simulink model "PubIfDecisionTOS_MDL"  (R2020b)
settings: configuration reference "DspaceConfig" (kept outside this file)
PostLoadFcn:
  | if any(exist('dsrtsu_mdlpostloadfcn', 'file') ~= 0), dsrtsu_mdlpostloadfcn('Execute', bdroot); end
InitFcn:
  | , if any(exist('dsmpb_private', 'file') ~= 0), dsmpb_private('dsmpb_mdlclblib', 'Init', bdroot); end,
undefined symbols (not defined in the file or in its folder): C_TOS_ACCEgoRAxletoFbumplength_m, C_TOS_ACCTargetFront_Flag, C_TOS_AEBJAPedObjDxThre_Val, C_TOS_AEBJAPedObjDyThre_Val, C_TOS_AEBJATargetSize_Val, C_TOS_AEBJAVehObjDxThre_Val, C_TOS_AEBJAVehObjDyThre_Val, C_TOS_AEBJuncPedTargetSize_Val, C_TOS_AEBLatObjDxThre_Val, C_TOS_AEBLatPedDyThre_Val, C_TOS_AEBLatTargetSize_Val, C_TOS_AEBLongTargetInEgoFront_Flag, C_TOS_axAbsGround_Parameter, C_TOS_CameraConfirmedFlag, C_TOS_CNsubjWidth, C_TOS_CurrentLaneCoreMinWidth_Val, C_TOS_CutInProb_Val_Zero, C_TOS_CutOutProb_Val_Zero, C_TOS_D2R_Val, C_TOS_DefaultValueObjectToCenterLine_dy, C_TOS_EgoCarWidth_Val, C_TOS_EgoDxRefPoint_m, C_TOS_EgoRAxletoFbumplength_m, C_TOS_HalfWidthVehicle_Con, C_TOS_HWA_CurrentLaneFlag, C_TOS_HWA_LeftLaneFlag, C_TOS_HWA_MovingDir_Vaild, C_TOS_HWA_MovState_Vaild, C_TOS_HWA_RightLaneFlag, C_TOS_LaneLineCourseErrorFront, C_TOS_LaneLineCourseErrorRear, C_TOS_MotorbikeDefaultWidth_m, C_TOS_NumberOfEffectiveTargets, C_TOS_Obj_Age_Val, C_TOS_Objdx_Constraint_Val, C_TOS_ObjectDefaultWidth_m, C_TOS_ObjInCurrentLane_Val, C_TOS_ObjInCurrentLaneValid, C_TOS_ObjInLeftLaneValid, C_TOS_ObjInRightLaneValid, C_TOS_ObjNotInCurrentLane_Val, C_TOS_ObjNotREElementType, C_TOS_ObjPredictDis_dy_ConstantVal_Zeros, C_TOS_ObjToCenterLine_ConstantVal_Zeros, C_TOS_OFMObjIDInvilad_Val, C_TOS_PIL_LatDisCons_Val_zero, C_TOS_PIL_ObjectCutInFlag_b, C_TOS_PIL_ObjectCutOutFlag_b, C_TOS_PIL_ObjLaneProb_al_Val, C_TOS_PP_ObjFusType_FC_Confirm_b, C_TOS_PP_ObjFusType_FC_FR_Confirm_b, C_TOS_PP_ObjFusType_FR_Confirm_b, C_TOS_RE_80BoolDefault_Val, C_TOS_RE_80Single181Default_Val, C_TOS_RE_80Single255Default_Val, C_TOS_RE_80Uint8Default_Val, C_TOS_RE_D2R, C_TOS_RE_D_180_Val, C_TOS_RE_InvalidObjectID_Val, C_TOS_RE_InvalidTargetChainDir_Val ... (+142)
libraries: simulink x1650, TOS_LIB x361, canfdmsglib x14
(part 46 of 69)

== system PubIfDecisionTOS_MDL/TOS_20201112/TOS_2012080320/TOS/AEB/TOS_AEBJunct1105/AEBJunc_Object_Condition/AEBJA_TargetCondition/TOS_AEBJunc_TargetsCondition/AEBJunc_VehTargetCondition/AEBJunc_VehTargetObjectTypeFlag ==
  ObjectType : Inport
  AEBJunc_VehTarget_ID_K1 : Inport  Port=2
  ObjectID : Inport  Port=3
  AEBJunc_VehTargetObjectTypeAborDly : Subsystem
  Compare To Constant3 : simulink/Logic and Bit Operations/Compare To Constant  relop===  const=OFM_OBJ_TYPE_E.CAR  OutDataTypeStr=boolean
      settings: AttributesFormatString=%<const>
  Compare To Constant4 : simulink/Logic and Bit Operations/Compare To Constant  relop===  const=OFM_OBJ_TYPE_E.TRUCK  OutDataTypeStr=boolean
      settings: AttributesFormatString=%<const>
  Data Type Conversion : DataTypeConversion  OutDataTypeStr=Enum: OFM_OBJ_TYPE_E
  Logical Operator3 : Logic  Operator=OR  AllPortsSameDT=off  OutDataTypeStr=boolean
  AEBJunc_VehTargetObjectTypeFlag : Outport
  wires:
  Logical Operator3/1 -> AEBJunc_VehTargetObjectTypeAborDly/3(TOS_AEBJunc_VehObjectType)
  ObjectType/1 -> Data Type Conversion/1
  Data Type Conversion/1 -> Compare To Constant3/1, Compare To Constant4/1
  Compare To Constant3/1 -> Logical Operator3/1
  Compare To Constant4/1 -> Logical Operator3/2
  AEBJunc_VehTarget_ID_K1/1 -> AEBJunc_VehTargetObjectTypeAborDly/1(AEBJunc_VehTarget_ID_K1)
  ObjectID/1 -> AEBJunc_VehTargetObjectTypeAborDly/2(ObjectID)
  AEBJunc_VehTargetObjectTypeAborDly/1(TOS_AEBJunc_VehObjectTypeFilt) -> AEBJunc_VehTargetObjectTypeFlag/1

== system PubIfDecisionTOS_MDL/TOS_20201112/TOS_2012080320/TOS/AEB/TOS_AEBJunct1105/AEBJunc_Object_Condition/AEBJA_TargetCondition/TOS_AEBJunc_TargetsCondition/AEBJunc_VehTargetCondition/Subsystem ==
  Object_MovingState : Inport
  Compare To Constant1 : simulink/Logic and Bit Operations/Compare To Constant  relop===  const=OFM_OBJ_MOVINGSTATE_E.MOVING  OutDataTypeStr=boolean
      settings: AttributesFormatString=%<const> = 2
  Compare To Constant2 : simulink/Logic and Bit Operations/Compare To Constant  relop===  const=OFM_OBJ_MOVINGSTATE_E.MOVING_SLOWLY  OutDataTypeStr=boolean
      settings: AttributesFormatString=%<const> = 5
  Data Type Conversion : DataTypeConversion  OutDataTypeStr=Enum: OFM_OBJ_MOVINGSTATE_E
  Logical Operator1 : Logic  Operator=OR  AllPortsSameDT=off  OutDataTypeStr=boolean
  TOS_AEBJuncVehTargetMovStateFlg : Outport
  wires:
  Compare To Constant1/1 -> Logical Operator1/1
  Logical Operator1/1 -> TOS_AEBJuncVehTargetMovStateFlg/1
  Compare To Constant2/1 -> Logical Operator1/2
  Object_MovingState/1 -> Data Type Conversion/1
  Data Type Conversion/1 -> Compare To Constant2/1, Compare To Constant1/1

== system PubIfDecisionTOS_MDL/TOS_20201112/TOS_2012080320/TOS/AEB/TOS_AEBJunct1105/AEBJunc_Object_Condition/AEBJA_TargetCondition/TOS_AEBJunc_TargetsCondition/AEBJunc_VehTargetCondition/TOS_AEBJunc_VehTargetMoveDir ==
  Object_Dx : Inport
  PP_ObjMovingDirSignalProcessing : Inport  Port=2
  Object_HeadingAngle : Inport  Port=3
  Object_VX : Inport  Port=4
  Object_VY : Inport  Port=5
  VIE_EgoVelocity : Inport  Port=6
  axvRefMs2 : Inport  Port=7
  Abs{,1..3} (4 alike) : Abs
  Add{,2..4} (4 alike) : Sum
  Add1 : Sum  Inputs=+-
  Compare To Constant : simulink/Logic and Bit Operations/Compare To Constant  relop=<  const=P_TOS_OncomingTarget_VxabsOffset_val  OutDataTypeStr=boolean
      settings: AttributesFormatString=%<const> = -0.7m/s
  Compare To Constant1 : simulink/Logic and Bit Operations/Compare To Constant  relop=>  const=P_TOS_CrossingTargetVyvThre_val  OutDataTypeStr=boolean
      settings: AttributesFormatString=%<const>
  Compare To Constant16 : simulink/Logic and Bit Operations/Compare To Constant  relop=>  const=P_TOS_ObjLatCroYawAngMaxThre_Val  OutDataTypeStr=boolean
      settings: AttributesFormatString=P_TOS_ObjLatCroYawAngMaxThre_Val = 135
  Compare To Constant2 : simulink/Logic and Bit Operations/Compare To Constant  relop===  const=ObjectMovingOrientation_E.OnComingDir  OutDataTypeStr=boolean
      settings: AttributesFormatString=%<const>
  Compare To Constant3 : simulink/Logic and Bit Operations/Compare To Constant  relop=>  const=P_TOS_ObjOncomingYawAngMaxThre_Val  OutDataTypeStr=boolean
      settings: AttributesFormatString=P_TOS_ObjOncomingYawAngMaxThre_Val = 180
  Compare To Constant4 : simulink/Logic and Bit Operations/Compare To Constant  relop=<  const=0  OutDataTypeStr=boolean
  Constant : Constant  Value=C_TOS_StepTime_Val
  Constant1 : Constant  Value=C_TOS_StepTime_Val
  Constant2 : Constant  Value=P_TOS_OncomingVehDxChangeOffset_Val
  Data Type Conversion2 : DataTypeConversion  OutDataTypeStr=Enum: ObjectMovingOrientation_E
  Gain : Gain  Gain=1/2
  Gain1 : Gain  Gain=1/2
  Logical Operator : Logic  Operator=OR  Inputs=4  AllPortsSameDT=off  OutDataTypeStr=boolean
  Logical Operator{1..3,10} (4 alike) : Logic  AllPortsSameDT=off  OutDataTypeStr=boolean
  Math Function : Math  Operator=square  SaturateOnIntegerOverflow=on
  Product : Product
  Product1 : Product
  Relational Operator : RelationalOperator  Operator=>  OutDataTypeStr=boolean  RndMeth=Simplest
  Unit Delay{,1..3} (4 alike) : UnitDelay  InitialCondition=255  SampleTime=-1  HasFrameUpgradeWarning=on
  TOS_AEBJuncVehTargetMovDirFlg : Outport
  wires:
  Logical Operator/1 -> TOS_AEBJuncVehTargetMovDirFlg/1
  VIE_EgoVelocity/1 -> [VIE_EgoVelocity], Add/2
  Logical Operator1/1 -> Logical Operator/3
  Abs2/1 -> Compare To Constant1/1
  PP_ObjMovingDirSignalProcessing/1 -> Data Type Conversion2/1
  Compare To Constant/1 -> Logical Operator1/1
  Abs1/1 -> Compare To Constant/1
  Data Type Conversion2/1 -> Compare To Constant2/1
  Abs/1 -> Compare To Constant16/1, Compare To Constant3/1
  Compare To Constant1/1 -> Logical Operator1/2
  Add/1 -> Abs1/1
  Logical Operator10/1 -> Logical Operator/2
  Compare To Constant16/1 -> Logical Operator10/1
  Object_VX/1 -> Add/1
  Compare To Constant2/1 -> Logical Operator/1
  Object_HeadingAngle/1 -> Abs/1
  Compare To Constant3/1 -> Logical Operator10/2
  Object_Dx/1 -> Add1/1, Unit Delay/1
  Unit Delay/1 -> Add1/2
  Add1/1 -> Compare To Constant4/1, Abs3/1
  Compare To Constant4/1 -> Logical Operator2/1
  Object_VY/1 -> Abs2/1
  Abs3/1 -> Relational Operator/1
  [VIE_EgoVelocity] -> Unit Delay2/1
  Constant/1 -> Product/2
  Constant1/1 -> Math Function/1
  Math Function/1 -> Product1/2
  Product1/1 -> Gain/1
  Gain/1 -> Add2/2
  Product/1 -> Add2/1
  axvRefMs2/1 -> Add3/1, Unit Delay1/1
  Add2/1 -> Add4/1
  Relational Operator/1 -> Unit Delay3/1, Logical Operator3/1
  Logical Operator2/1 -> Logical Operator/4
  Unit Delay1/1 -> Add3/2
  Add3/1 -> Gain1/1
  Gain1/1 -> Product1/1
  Unit Delay2/1 -> Product/1
  Constant2/1 -> Add4/2
  Add4/1 -> Relational Operator/2
  Unit Delay3/1 -> Logical Operator3/2
  Logical Operator3/1 -> Logical Operator2/2

== system PubIfDecisionTOS_MDL/TOS_20201112/TOS_2012080320/TOS/AEB/TOS_AEBJunct1105/AEBJunc_Object_Condition1/AEBJA_TargetCondition/TOS_AEBJunc_TargetsCondition/AEBJunc_PedTargetCondition/AEBJunc_PedTargetADxDyArea ==
  Object_Dx : Inport
  Object_Dy : Inport  Port=2
  Abs : Abs
  Compare To Constant1 : simulink/Logic and Bit Operations/Compare To Constant  relop=<=  const=C_TOS_AEBJAPedObjDxThre_Val  OutDataTypeStr=boolean
      settings: AttributesFormatString=C_TOS_AEBJAObjDxThre_Val = 25
  Compare To Constant2 : simulink/Logic and Bit Operations/Compare To Constant  relop=>  const=C_TOS_EgoDxRefPoint_m  OutDataTypeStr=boolean
      settings: AttributesFormatString=C_TOS_EgoDxRefPoint_m = 0
  Compare To Constant6 : simulink/Logic and Bit Operations/Compare To Constant  relop=<=  const=C_TOS_AEBJAPedObjDyThre_Val  OutDataTypeStr=boolean
      settings: AttributesFormatString=C_TOS_AEBJAObjDyThre_Val = 10 m
  Logical Operator : Logic  AllPortsSameDT=off  OutDataTypeStr=boolean
  Logical Operator1 : Logic  AllPortsSameDT=off  OutDataTypeStr=boolean
  TOS_AEBJunc_DxDyAreaFlag : Outport
  wires:
  Object_Dx/1 -> Compare To Constant2/1, Compare To Constant1/1
  Compare To Constant6/1 -> Logical Operator1/2
  Logical Operator1/1 -> TOS_AEBJunc_DxDyAreaFlag/1
  Compare To Constant2/1 -> Logical Operator/2
  Compare To Constant1/1 -> Logical Operator/1
  Abs/1 -> Compare To Constant6/1
  Object_Dy/1 -> Abs/1
  Logical Operator/1 -> Logical Operator1/1

== system PubIfDecisionTOS_MDL/TOS_20201112/TOS_2012080320/TOS/AEB/TOS_AEBJunct1105/AEBJunc_Object_Condition1/AEBJA_TargetCondition/TOS_AEBJunc_TargetsCondition/AEBJunc_PedTargetCondition/AEBJunc_PedTargetFusionTypeJudge ==
  PP_ObjFusType_FC_FR_Confirm : Inport
  PP_ObjFusType_FR_Confirm : Inport  Port=2
  Compare To Constant5 : simulink/Logic and Bit Operations/Compare To Constant  relop===  const=C_TOS_PP_ObjFusType_FC_FR_Confirm_b  OutDataTypeStr=boolean
      settings: AttributesFormatString=C_TOS_PP_ObjFusType_FC_FR_Confirm_b = 1
  Compare To Constant6 : simulink/Logic and Bit Operations/Compare To Constant  relop===  const=C_TOS_PP_ObjFusType_FR_Confirm_b  OutDataTypeStr=boolean
      settings: AttributesFormatString=C_TOS_PP_ObjFusType_FR_Confirm_b = 1
  Logical Operator : Logic  Operator=OR  AllPortsSameDT=off  OutDataTypeStr=boolean
  AEBJunc_TargetFusionTypeFlag : Outport
  wires:
  Logical Operator/1 -> AEBJunc_TargetFusionTypeFlag/1
  Compare To Constant5/1 -> Logical Operator/1
  Compare To Constant6/1 -> Logical Operator/2
  PP_ObjFusType_FC_FR_Confirm/1 -> Compare To Constant5/1
  PP_ObjFusType_FR_Confirm/1 -> Compare To Constant6/1

== system PubIfDecisionTOS_MDL/TOS_20201112/TOS_2012080320/TOS/AEB/TOS_AEBJunct1105/AEBJunc_Object_Condition1/AEBJA_TargetCondition/TOS_AEBJunc_TargetsCondition/AEBJunc_PedTargetCondition/AEBJunc_PedTargetMoveDir ==
  Object_Dy : Inport
  Object_Dx : Inport  Port=2
  PP_ObjMovingDirSignalProcessing : Inport  Port=3
  Object_HeadingAngle : Inport  Port=4
  Object_VX : Inport  Port=5
  Object_VY : Inport  Port=6
  VIE_EgoVelocity : Inport  Port=7
  axvRefMs2 : Inport  Port=8
  Bus Creator : BusCreator  Inputs=8
  Logical Operator : Logic  Operator=OR  AllPortsSameDT=off  OutDataTypeStr=boolean
  TOS_AEBJuncTargetCrossing : Subsystem
  TOS_AEBJuncTargetOncoming : Subsystem
  TOS_AEBJuncTargetMovDirFlg : Outport
  wires:
  Logical Operator/1 -> TOS_AEBJuncTargetMovDirFlg/1
  axvRefMs2/1 -> Bus Creator/8  "axvRefMs2"
  Object_Dx/1 -> Bus Creator/2  "Object_Dx"
  TOS_AEBJuncTargetOncoming/1(TOS_AEBJuncTargetOncomingFlg) -> Logical Operator/2
  TOS_AEBJuncTargetCrossing/1(TOS_AEBJuncTargetCrossingFlg) -> Logical Operator/1
  Bus Creator/1 -> TOS_AEBJuncTargetCrossing/1(Object_Infor), TOS_AEBJuncTargetOncoming/1(Object_Infor)
  Object_Dy/1 -> Bus Creator/1  "Object_Dy"
  Object_VY/1 -> Bus Creator/6  "Object_VY"
  VIE_EgoVelocity/1 -> Bus Creator/7  "VIE_EgoVelocity"
  Object_VX/1 -> Bus Creator/5  "Object_VX"
  Object_HeadingAngle/1 -> Bus Creator/4  "Object_HeadingAngle"
  PP_ObjMovingDirSignalProcessing/1 -> Bus Creator/3  "PP_ObjMovingDirSignalProcessing"

== system PubIfDecisionTOS_MDL/TOS_20201112/TOS_2012080320/TOS/AEB/TOS_AEBJunct1105/AEBJunc_Object_Condition1/AEBJA_TargetCondition/TOS_AEBJunc_TargetsCondition/AEBJunc_PedTargetCondition/AEBJunc_PedTargetObjectTypeFlag ==
  ObjectType : Inport
  AEBLat_Target_ID_K1 : Inport  Port=2
  ObjectID : Inport  Port=3
  AEBJunc_PedTargetObjectTypeAborDly : Subsystem
  Compare To Constant3 : simulink/Logic and Bit Operations/Compare To Constant  relop===  const=OFM_OBJ_TYPE_E.PEDESTRIAN  OutDataTypeStr=boolean
      settings: AttributesFormatString=%<const>
  Compare To Constant4 : simulink/Logic and Bit Operations/Compare To Constant  relop===  const=OFM_OBJ_TYPE_E.MOTORBIKE  OutDataTypeStr=boolean
      settings: AttributesFormatString=%<const>
  Compare To Constant5 : simulink/Logic and Bit Operations/Compare To Constant  relop===  const=OFM_OBJ_TYPE_E.BICYCLE  OutDataTypeStr=boolean
      settings: AttributesFormatString=%<const>
  Data Type Conversion : DataTypeConversion  OutDataTypeStr=Enum: OFM_OBJ_TYPE_E
  Logical Operator3 : Logic  Operator=OR  Inputs=3  AllPortsSameDT=off  OutDataTypeStr=boolean
  AEBJunc_PedTargetObjectTypeFlag : Outport
  wires:
  AEBJunc_PedTargetObjectTypeAborDly/1(TOS_AEBJunc_PedObjectTypeFilt) -> AEBJunc_PedTargetObjectTypeFlag/1
  AEBLat_Target_ID_K1/1 -> AEBJunc_PedTargetObjectTypeAborDly/1(AEBJunc_PedTarget_ID_K1)
  ObjectID/1 -> AEBJunc_PedTargetObjectTypeAborDly/2(ObjectID)
  Compare To Constant3/1 -> Logical Operator3/1
  Compare To Constant5/1 -> Logical Operator3/3
  Compare To Constant4/1 -> Logical Operator3/2
  Logical Operator3/1 -> AEBJunc_PedTargetObjectTypeAborDly/3(TOS_AEBJunc_PedObjectType)
  ObjectType/1 -> Data Type Conversion/1
  Data Type Conversion/1 -> Compare To Constant4/1, Compare To Constant5/1, Compare To Constant3/1

== system PubIfDecisionTOS_MDL/TOS_20201112/TOS_2012080320/TOS/AEB/TOS_AEBJunct1105/AEBJunc_Object_Condition1/AEBJA_TargetCondition/TOS_AEBJunc_TargetsCondition/AEBJunc_VehTargetCondition/AEBJunc_VehTargetADxDyArea ==
  Object_Dx : Inport
  Object_Dy : Inport  Port=2
  Abs : Abs
  Compare To Constant1 : simulink/Logic and Bit Operations/Compare To Constant  relop=<=  const=C_TOS_AEBJAVehObjDxThre_Val  OutDataTypeStr=boolean
      settings: AttributesFormatString=%<const> = 50
  Compare To Constant2 : simulink/Logic and Bit Operations/Compare To Constant  relop=>  const=C_TOS_EgoDxRefPoint_m  OutDataTypeStr=boolean
      settings: AttributesFormatString=C_TOS_EgoDxRefPoint_m = 0
  Compare To Constant6 : simulink/Logic and Bit Operations/Compare To Constant  relop=<=  const=C_TOS_AEBJAVehObjDyThre_Val  OutDataTypeStr=boolean
      settings: AttributesFormatString=C_TOS_AEBJAVehObjDyThre_Val = 10 m
  Logical Operator : Logic  AllPortsSameDT=off  OutDataTypeStr=boolean
  Logical Operator1 : Logic  AllPortsSameDT=off  OutDataTypeStr=boolean
  TOS_AEBJunc_VehDxDyAreaFlag : Outport
  wires:
  Logical Operator/1 -> Logical Operator1/1
  Object_Dy/1 -> Abs/1
  Abs/1 -> Compare To Constant6/1
  Compare To Constant1/1 -> Logical Operator/1
  Compare To Constant2/1 -> Logical Operator/2
  Logical Operator1/1 -> TOS_AEBJunc_VehDxDyAreaFlag/1
  Compare To Constant6/1 -> Logical Operator1/2
  Object_Dx/1 -> Compare To Constant1/1, Compare To Constant2/1

== system PubIfDecisionTOS_MDL/TOS_20201112/TOS_2012080320/TOS/AEB/TOS_AEBJunct1105/AEBJunc_Object_Condition1/AEBJA_TargetCondition/TOS_AEBJunc_TargetsCondition/AEBJunc_VehTargetCondition/AEBJunc_VehTargetFusionTypeJudge ==
  PP_ObjFusType_FC_FR_Confirm : Inport
  PP_ObjFusType_FR_Confirm : Inport  Port=2
  Compare To Constant5 : simulink/Logic and Bit Operations/Compare To Constant  relop===  const=C_TOS_PP_ObjFusType_FC_FR_Confirm_b  OutDataTypeStr=boolean
      settings: AttributesFormatString=C_TOS_PP_ObjFusType_FC_FR_Confirm_b = 1
  Compare To Constant6 : simulink/Logic and Bit Operations/Compare To Constant  relop===  const=C_TOS_PP_ObjFusType_FR_Confirm_b  OutDataTypeStr=boolean
      settings: AttributesFormatString=C_TOS_PP_ObjFusType_FR_Confirm_b = 1
  Logical Operator : Logic  Operator=OR  AllPortsSameDT=off  OutDataTypeStr=boolean
  AEBJunc_VehTargetFusionTypeFlag : Outport
  wires:
  PP_ObjFusType_FR_Confirm/1 -> Compare To Constant6/1
  PP_ObjFusType_FC_FR_Confirm/1 -> Compare To Constant5/1
  Compare To Constant6/1 -> Logical Operator/2
  Compare To Constant5/1 -> Logical Operator/1
  Logical Operator/1 -> AEBJunc_VehTargetFusionTypeFlag/1

== system PubIfDecisionTOS_MDL/TOS_20201112/TOS_2012080320/TOS/AEB/TOS_AEBJunct1105/AEBJunc_Object_Condition1/AEBJA_TargetCondition/TOS_AEBJunc_TargetsCondition/AEBJunc_VehTargetCondition/AEBJunc_VehTargetObjectTypeFlag ==
  ObjectType : Inport
  AEBJunc_VehTarget_ID_K1 : Inport  Port=2
  ObjectID : Inport  Port=3
  AEBJunc_VehTargetObjectTypeAborDly : Subsystem
  Compare To Constant3 : simulink/Logic and Bit Operations/Compare To Constant  relop===  const=OFM_OBJ_TYPE_E.CAR  OutDataTypeStr=boolean
      settings: AttributesFormatString=%<const>
  Compare To Constant4 : simulink/Logic and Bit Operations/Compare To Constant  relop===  const=OFM_OBJ_TYPE_E.TRUCK  OutDataTypeStr=boolean
      settings: AttributesFormatString=%<const>
  Data Type Conversion : DataTypeConversion  OutDataTypeStr=Enum: OFM_OBJ_TYPE_E
  Logical Operator3 : Logic  Operator=OR  AllPortsSameDT=off  OutDataTypeStr=boolean
  AEBJunc_VehTargetObjectTypeFlag : Outport
  wires:
  AEBJunc_VehTargetObjectTypeAborDly/1(TOS_AEBJunc_VehObjectTypeFilt) -> AEBJunc_VehTargetObjectTypeFlag/1
  ObjectID/1 -> AEBJunc_VehTargetObjectTypeAborDly/2(ObjectID)
  AEBJunc_VehTarget_ID_K1/1 -> AEBJunc_VehTargetObjectTypeAborDly/1(AEBJunc_VehTarget_ID_K1)
  Compare To Constant4/1 -> Logical Operator3/2
  Compare To Constant3/1 -> Logical Operator3/1
  Data Type Conversion/1 -> Compare To Constant4/1, Compare To Constant3/1
  ObjectType/1 -> Data Type Conversion/1
  Logical Operator3/1 -> AEBJunc_VehTargetObjectTypeAborDly/3(TOS_AEBJunc_VehObjectType)

== system PubIfDecisionTOS_MDL/TOS_20201112/TOS_2012080320/TOS/AEB/TOS_AEBJunct1105/AEBJunc_Object_Condition1/AEBJA_TargetCondition/TOS_AEBJunc_TargetsCondition/AEBJunc_VehTargetCondition/Subsystem ==
  Object_MovingState : Inport
  Compare To Constant1 : simulink/Logic and Bit Operations/Compare To Constant  relop===  const=OFM_OBJ_MOVINGSTATE_E.MOVING  OutDataTypeStr=boolean
      settings: AttributesFormatString=%<const> = 2
  Compare To Constant2 : simulink/Logic and Bit Operations/Compare To Constant  relop===  const=OFM_OBJ_MOVINGSTATE_E.MOVING_SLOWLY  OutDataTypeStr=boolean
      settings: AttributesFormatString=%<const> = 5
  Data Type Conversion : DataTypeConversion  OutDataTypeStr=Enum: OFM_OBJ_MOVINGSTATE_E
  Logical Operator1 : Logic  Operator=OR  AllPortsSameDT=off  OutDataTypeStr=boolean
  TOS_AEBJuncVehTargetMovStateFlg : Outport
  wires:
  Data Type Conversion/1 -> Compare To Constant1/1, Compare To Constant2/1
  Object_MovingState/1 -> Data Type Conversion/1
  Compare To Constant2/1 -> Logical Operator1/2
  Logical Operator1/1 -> TOS_AEBJuncVehTargetMovStateFlg/1
  Compare To Constant1/1 -> Logical Operator1/1

== system PubIfDecisionTOS_MDL/TOS_20201112/TOS_2012080320/TOS/AEB/TOS_AEBJunct1105/AEBJunc_Object_Condition1/AEBJA_TargetCondition/TOS_AEBJunc_TargetsCondition/AEBJunc_VehTargetCondition/TOS_AEBJunc_VehTargetMoveDir ==
  Object_Dx : Inport
  PP_ObjMovingDirSignalProcessing : Inport  Port=2
  Object_HeadingAngle : Inport  Port=3
  Object_VX : Inport  Port=4
  Object_VY : Inport  Port=5
  VIE_EgoVelocity : Inport  Port=6
  axvRefMs2 : Inport  Port=7
  Abs{,1..3} (4 alike) : Abs
  Add{,2..4} (4 alike) : Sum
  Add1 : Sum  Inputs=+-
  Compare To Constant : simulink/Logic and Bit Operations/Compare To Constant  relop=<  const=P_TOS_OncomingTarget_VxabsOffset_val  OutDataTypeStr=boolean
      settings: AttributesFormatString=%<const> = -0.7m/s
  Compare To Constant1 : simulink/Logic and Bit Operations/Compare To Constant  relop=>  const=P_TOS_CrossingTargetVyvThre_val  OutDataTypeStr=boolean
      settings: AttributesFormatString=%<const>
  Compare To Constant16 : simulink/Logic and Bit Operations/Compare To Constant  relop=>  const=P_TOS_ObjLatCroYawAngMaxThre_Val  OutDataTypeStr=boolean
      settings: AttributesFormatString=P_TOS_ObjLatCroYawAngMaxThre_Val = 135
  Compare To Constant2 : simulink/Logic and Bit Operations/Compare To Constant  relop===  const=ObjectMovingOrientation_E.OnComingDir  OutDataTypeStr=boolean
      settings: AttributesFormatString=%<const>
  Compare To Constant3 : simulink/Logic and Bit Operations/Compare To Constant  relop=>  const=P_TOS_ObjOncomingYawAngMaxThre_Val  OutDataTypeStr=boolean
      settings: AttributesFormatString=P_TOS_ObjOncomingYawAngMaxThre_Val = 180
  Compare To Constant4 : simulink/Logic and Bit Operations/Compare To Constant  relop=<  const=0  OutDataTypeStr=boolean
  Constant : Constant  Value=C_TOS_StepTime_Val
  Constant1 : Constant  Value=C_TOS_StepTime_Val
  Constant2 : Constant  Value=P_TOS_OncomingVehDxChangeOffset_Val
  Data Type Conversion2 : DataTypeConversion  OutDataTypeStr=Enum: ObjectMovingOrientation_E
  Gain : Gain  Gain=1/2
  Gain1 : Gain  Gain=1/2
  Logical Operator : Logic  Operator=OR  Inputs=4  AllPortsSameDT=off  OutDataTypeStr=boolean
  Logical Operator{1..3,10} (4 alike) : Logic  AllPortsSameDT=off  OutDataTypeStr=boolean
  Math Function : Math  Operator=square  SaturateOnIntegerOverflow=on
  Product : Product
  Product1 : Product
  Relational Operator : RelationalOperator  Operator=>  OutDataTypeStr=boolean  RndMeth=Simplest
  Unit Delay{,1..3} (4 alike) : UnitDelay  InitialCondition=255  SampleTime=-1  HasFrameUpgradeWarning=on
  TOS_AEBJuncVehTargetMovDirFlg : Outport
  wires:
  Logical Operator3/1 -> Logical Operator2/2
  Unit Delay3/1 -> Logical Operator3/2
  Add4/1 -> Relational Operator/2
  Constant2/1 -> Add4/2
  Unit Delay2/1 -> Product/1
  Gain1/1 -> Product1/1
  Add3/1 -> Gain1/1
  Unit Delay1/1 -> Add3/2
  Logical Operator2/1 -> Logical Operator/4
  Relational Operator/1 -> Logical Operator3/1, Unit Delay3/1
  Add2/1 -> Add4/1
  axvRefMs2/1 -> Unit Delay1/1, Add3/1
  Product/1 -> Add2/1
  Gain/1 -> Add2/2
  Product1/1 -> Gain/1
  Math Function/1 -> Product1/2
  Constant1/1 -> Math Function/1
  Constant/1 -> Product/2
  [VIE_EgoVelocity] -> Unit Delay2/1
  Abs3/1 -> Relational Operator/1
  Object_VY/1 -> Abs2/1
  Compare To Constant4/1 -> Logical Operator2/1
  Add1/1 -> Abs3/1, Compare To Constant4/1
  Unit Delay/1 -> Add1/2
  Object_Dx/1 -> Unit Delay/1, Add1/1
  Compare To Constant3/1 -> Logical Operator10/2
  Object_HeadingAngle/1 -> Abs/1
  Compare To Constant2/1 -> Logical Operator/1
  Object_VX/1 -> Add/1
  Compare To Constant16/1 -> Logical Operator10/1
  Logical Operator10/1 -> Logical Operator/2
  Add/1 -> Abs1/1
  Compare To Constant1/1 -> Logical Operator1/2
  Abs/1 -> Compare To Constant3/1, Compare To Constant16/1
  Data Type Conversion2/1 -> Compare To Constant2/1
  Abs1/1 -> Compare To Constant/1
  Compare To Constant/1 -> Logical Operator1/1
  PP_ObjMovingDirSignalProcessing/1 -> Data Type Conversion2/1
  Abs2/1 -> Compare To Constant1/1
  Logical Operator1/1 -> Logical Operator/3
  VIE_EgoVelocity/1 -> Add/2, [VIE_EgoVelocity]
  Logical Operator/1 -> TOS_AEBJuncVehTargetMovDirFlg/1

== system PubIfDecisionTOS_MDL/TOS_20201112/TOS_2012080320/TOS/AEB/TOS_AEBJunct_20201208/AEBJunc_Object_Condition/AEBJA_TargetCondition/TOS_AEBJunc_TargetsCondition/AEBJunc_PedTargetCondition/AEBJunc_PedTargetADxDyArea ==
  Object_Dx : Inport
  Object_Dy : Inport  Port=2
  Abs : Abs
  Compare To Constant1 : simulink/Logic and Bit Operations/Compare To Constant  relop=<=  const=C_TOS_AEBJAPedObjDxThre_Val  OutDataTypeStr=boolean
      settings: AttributesFormatString=C_TOS_AEBJAObjDxThre_Val = 25
  Compare To Constant2 : simulink/Logic and Bit Operations/Compare To Constant  relop=>  const=C_TOS_EgoDxRefPoint_m  OutDataTypeStr=boolean
      settings: AttributesFormatString=C_TOS_EgoDxRefPoint_m = 0
  Compare To Constant6 : simulink/Logic and Bit Operations/Compare To Constant  relop=<=  const=C_TOS_AEBJAPedObjDyThre_Val  OutDataTypeStr=boolean
      settings: AttributesFormatString=C_TOS_AEBJAObjDyThre_Val = 10 m
  Logical Operator : Logic  AllPortsSameDT=off  OutDataTypeStr=boolean
  Logical Operator1 : Logic  AllPortsSameDT=off  OutDataTypeStr=boolean
  TOS_AEBJunc_DxDyAreaFlag : Outport
  wires:
  Logical Operator/1 -> Logical Operator1/1
  Object_Dy/1 -> Abs/1
  Abs/1 -> Compare To Constant6/1
  Compare To Constant1/1 -> Logical Operator/1
  Compare To Constant2/1 -> Logical Operator/2
  Logical Operator1/1 -> TOS_AEBJunc_DxDyAreaFlag/1
  Compare To Constant6/1 -> Logical Operator1/2
  Object_Dx/1 -> Compare To Constant1/1, Compare To Constant2/1

== system PubIfDecisionTOS_MDL/TOS_20201112/TOS_2012080320/TOS/AEB/TOS_AEBJunct_20201208/AEBJunc_Object_Condition/AEBJA_TargetCondition/TOS_AEBJunc_TargetsCondition/AEBJunc_PedTargetCondition/AEBJunc_PedTargetFusionTypeJudge ==
  PP_ObjFusType_FC_FR_Confirm : Inport
  PP_ObjFusType_FR_Confirm : Inport  Port=2
  Compare To Constant5 : simulink/Logic and Bit Operations/Compare To Constant  relop===  const=C_TOS_PP_ObjFusType_FC_FR_Confirm_b  OutDataTypeStr=boolean
      settings: AttributesFormatString=C_TOS_PP_ObjFusType_FC_FR_Confirm_b = 1
  Compare To Constant6 : simulink/Logic and Bit Operations/Compare To Constant  relop===  const=C_TOS_PP_ObjFusType_FR_Confirm_b  OutDataTypeStr=boolean
      settings: AttributesFormatString=C_TOS_PP_ObjFusType_FR_Confirm_b = 1
  Logical Operator : Logic  Operator=OR  AllPortsSameDT=off  OutDataTypeStr=boolean
  AEBJunc_TargetFusionTypeFlag : Outport
  wires:
  PP_ObjFusType_FR_Confirm/1 -> Compare To Constant6/1
  PP_ObjFusType_FC_FR_Confirm/1 -> Compare To Constant5/1
  Compare To Constant6/1 -> Logical Operator/2
  Compare To Constant5/1 -> Logical Operator/1
  Logical Operator/1 -> AEBJunc_TargetFusionTypeFlag/1

== system PubIfDecisionTOS_MDL/TOS_20201112/TOS_2012080320/TOS/AEB/TOS_AEBJunct_20201208/AEBJunc_Object_Condition/AEBJA_TargetCondition/TOS_AEBJunc_TargetsCondition/AEBJunc_PedTargetCondition/AEBJunc_PedTargetMoveDir ==
  Object_Dy : Inport
  Object_Dx : Inport  Port=2
  PP_ObjMovingDirSignalProcessing : Inport  Port=3
  Object_HeadingAngle : Inport  Port=4
  Object_VX : Inport  Port=5
  Object_VY : Inport  Port=6
  VIE_EgoVelocity : Inport  Port=7
  axvRefMs2 : Inport  Port=8
  AEBJunc_Target_ID_K1 : Inport  Port=9
  ObjectID : Inport  Port=10
  AEBLat_TargetMovDirAborDly : Subsystem
  Bus Creator : BusCreator  Inputs=8
  Logical Operator : Logic  Operator=OR  AllPortsSameDT=off  OutDataTypeStr=boolean
  TOS_AEBJuncTargetCrossing : Subsystem
  TOS_AEBJuncTargetOncoming : Subsystem
  TOS_AEBJuncTargetMovDirFlg : Outport
  wires:
  PP_ObjMovingDirSignalProcessing/1 -> Bus Creator/3  "PP_ObjMovingDirSignalProcessing"
  Object_HeadingAngle/1 -> Bus Creator/4  "Object_HeadingAngle"
  Object_VX/1 -> Bus Creator/5  "Object_VX"
  VIE_EgoVelocity/1 -> Bus Creator/7  "VIE_EgoVelocity"
  Object_VY/1 -> Bus Creator/6  "Object_VY"
  Object_Dy/1 -> Bus Creator/1  "Object_Dy"
  Bus Creator/1 -> TOS_AEBJuncTargetOncoming/1(Object_Infor), TOS_AEBJuncTargetCrossing/1(Object_Infor)
  TOS_AEBJuncTargetCrossing/1(TOS_AEBJuncTargetCrossingFlg) -> Logical Operator/1
  TOS_AEBJuncTargetOncoming/1(TOS_AEBJuncTargetOncomingFlg) -> Logical Operator/2
  Object_Dx/1 -> Bus Creator/2  "Object_Dx"
  axvRefMs2/1 -> Bus Creator/8  "axvRefMs2"
  Logical Operator/1 -> AEBLat_TargetMovDirAborDly/3(TOS_AEBJunc_MovDir_Flag)
  AEBJunc_Target_ID_K1/1 -> AEBLat_TargetMovDirAborDly/1(AEBJunc_Target_ID_K1)
  ObjectID/1 -> AEBLat_TargetMovDirAborDly/2(ObjectID)
  AEBLat_TargetMovDirAborDly/1(TOS_AEBJunc_MovDirFlag_Delay) -> TOS_AEBJuncTargetMovDirFlg/1

== system PubIfDecisionTOS_MDL/TOS_20201112/TOS_2012080320/TOS/AEB/TOS_AEBJunct_20201208/AEBJunc_Object_Condition/AEBJA_TargetCondition/TOS_AEBJunc_TargetsCondition/AEBJunc_PedTargetCondition/AEBJunc_PedTargetObjectTypeFlag ==
  ObjectType : Inport
  AEBLat_Target_ID_K1 : Inport  Port=2
  ObjectID : Inport  Port=3
  AEBJunc_PedTargetObjectTypeAborDly : Subsystem
  Compare To Constant3 : simulink/Logic and Bit Operations/Compare To Constant  relop===  const=OFM_OBJ_TYPE_E.PEDESTRIAN  OutDataTypeStr=boolean
      settings: AttributesFormatString=%<const>
  Compare To Constant4 : simulink/Logic and Bit Operations/Compare To Constant  relop===  const=OFM_OBJ_TYPE_E.MOTORBIKE  OutDataTypeStr=boolean
      settings: AttributesFormatString=%<const>
  Compare To Constant5 : simulink/Logic and Bit Operations/Compare To Constant  relop===  const=OFM_OBJ_TYPE_E.BICYCLE  OutDataTypeStr=boolean
      settings: AttributesFormatString=%<const>
  Data Type Conversion : DataTypeConversion  OutDataTypeStr=Enum: OFM_OBJ_TYPE_E
  Logical Operator3 : Logic  Operator=OR  Inputs=3  AllPortsSameDT=off  OutDataTypeStr=boolean
  AEBJunc_PedTargetObjectTypeFlag : Outport
  wires:
  Data Type Conversion/1 -> Compare To Constant3/1, Compare To Constant5/1, Compare To Constant4/1
  ObjectType/1 -> Data Type Conversion/1
  Logical Operator3/1 -> AEBJunc_PedTargetObjectTypeAborDly/3(TOS_AEBJunc_PedObjectType)
  Compare To Constant4/1 -> Logical Operator3/2
  Compare To Constant5/1 -> Logical Operator3/3
  Compare To Constant3/1 -> Logical Operator3/1
  ObjectID/1 -> AEBJunc_PedTargetObjectTypeAborDly/2(ObjectID)
  AEBLat_Target_ID_K1/1 -> AEBJunc_PedTargetObjectTypeAborDly/1(AEBJunc_PedTarget_ID_K1)
  AEBJunc_PedTargetObjectTypeAborDly/1(TOS_AEBJunc_PedObjectTypeFilt) -> AEBJunc_PedTargetObjectTypeFlag/1

== system PubIfDecisionTOS_MDL/TOS_20201112/TOS_2012080320/TOS/AEB/TOS_AEBJunct_20201208/AEBJunc_Object_Condition/AEBJA_TargetCondition/TOS_AEBJunc_TargetsCondition/AEBJunc_VehTargetCondition/AEBJunc_VehTargetADxDyArea ==
  Object_Dx : Inport
  Object_Dy : Inport  Port=2
  Abs : Abs
  Compare To Constant1 : simulink/Logic and Bit Operations/Compare To Constant  relop=<=  const=C_TOS_AEBJAVehObjDxThre_Val  OutDataTypeStr=boolean
      settings: AttributesFormatString=%<const> = 50
  Compare To Constant2 : simulink/Logic and Bit Operations/Compare To Constant  relop=>  const=C_TOS_EgoDxRefPoint_m  OutDataTypeStr=boolean
      settings: AttributesFormatString=C_TOS_EgoDxRefPoint_m = 0
  Compare To Constant6 : simulink/Logic and Bit Operations/Compare To Constant  relop=<=  const=C_TOS_AEBJAVehObjDyThre_Val  OutDataTypeStr=boolean
      settings: AttributesFormatString=C_TOS_AEBJAVehObjDyThre_Val = 10 m
  Logical Operator : Logic  AllPortsSameDT=off  OutDataTypeStr=boolean
  Logical Operator1 : Logic  AllPortsSameDT=off  OutDataTypeStr=boolean
  TOS_AEBJunc_VehDxDyAreaFlag : Outport
  wires:
  Object_Dx/1 -> Compare To Constant2/1, Compare To Constant1/1
  Compare To Constant6/1 -> Logical Operator1/2
  Logical Operator1/1 -> TOS_AEBJunc_VehDxDyAreaFlag/1
  Compare To Constant2/1 -> Logical Operator/2
  Compare To Constant1/1 -> Logical Operator/1
  Abs/1 -> Compare To Constant6/1
  Object_Dy/1 -> Abs/1
  Logical Operator/1 -> Logical Operator1/1

== system PubIfDecisionTOS_MDL/TOS_20201112/TOS_2012080320/TOS/AEB/TOS_AEBJunct_20201208/AEBJunc_Object_Condition/AEBJA_TargetCondition/TOS_AEBJunc_TargetsCondition/AEBJunc_VehTargetCondition/AEBJunc_VehTargetFusionTypeJudge ==
  PP_ObjFusType_FC_FR_Confirm : Inport
  PP_ObjFusType_FR_Confirm : Inport  Port=2
  Compare To Constant5 : simulink/Logic and Bit Operations/Compare To Constant  relop===  const=C_TOS_PP_ObjFusType_FC_FR_Confirm_b  OutDataTypeStr=boolean
      settings: AttributesFormatString=C_TOS_PP_ObjFusType_FC_FR_Confirm_b = 1
  Compare To Constant6 : simulink/Logic and Bit Operations/Compare To Constant  relop===  const=C_TOS_PP_ObjFusType_FR_Confirm_b  OutDataTypeStr=boolean
      settings: AttributesFormatString=C_TOS_PP_ObjFusType_FR_Confirm_b = 1
  Logical Operator : Logic  Operator=OR  AllPortsSameDT=off  OutDataTypeStr=boolean
  AEBJunc_VehTargetFusionTypeFlag : Outport
  wires:
  Logical Operator/1 -> AEBJunc_VehTargetFusionTypeFlag/1
  Compare To Constant5/1 -> Logical Operator/1
  Compare To Constant6/1 -> Logical Operator/2
  PP_ObjFusType_FC_FR_Confirm/1 -> Compare To Constant5/1
  PP_ObjFusType_FR_Confirm/1 -> Compare To Constant6/1

== system PubIfDecisionTOS_MDL/TOS_20201112/TOS_2012080320/TOS/AEB/TOS_AEBJunct_20201208/AEBJunc_Object_Condition/AEBJA_TargetCondition/TOS_AEBJunc_TargetsCondition/AEBJunc_VehTargetCondition/AEBJunc_VehTargetObjectTypeFlag ==
  ObjectType : Inport
  AEBJunc_VehTarget_ID_K1 : Inport  Port=2
  ObjectID : Inport  Port=3
  AEBJunc_VehTargetObjectTypeAborDly : Subsystem
  Compare To Constant3 : simulink/Logic and Bit Operations/Compare To Constant  relop===  const=OFM_OBJ_TYPE_E.CAR  OutDataTypeStr=boolean
      settings: AttributesFormatString=%<const>
  Compare To Constant4 : simulink/Logic and Bit Operations/Compare To Constant  relop===  const=OFM_OBJ_TYPE_E.TRUCK  OutDataTypeStr=boolean
      settings: AttributesFormatString=%<const>
  Data Type Conversion : DataTypeConversion  OutDataTypeStr=Enum: OFM_OBJ_TYPE_E
  Logical Operator3 : Logic  Operator=OR  AllPortsSameDT=off  OutDataTypeStr=boolean
  AEBJunc_VehTargetObjectTypeFlag : Outport
  wires:
  Logical Operator3/1 -> AEBJunc_VehTargetObjectTypeAborDly/3(TOS_AEBJunc_VehObjectType)
  ObjectType/1 -> Data Type Conversion/1
  Data Type Conversion/1 -> Compare To Constant3/1, Compare To Constant4/1
  Compare To Constant3/1 -> Logical Operator3/1
  Compare To Constant4/1 -> Logical Operator3/2
  AEBJunc_VehTarget_ID_K1/1 -> AEBJunc_VehTargetObjectTypeAborDly/1(AEBJunc_VehTarget_ID_K1)
  ObjectID/1 -> AEBJunc_VehTargetObjectTypeAborDly/2(ObjectID)
  AEBJunc_VehTargetObjectTypeAborDly/1(TOS_AEBJunc_VehObjectTypeFilt) -> AEBJunc_VehTargetObjectTypeFlag/1

== system PubIfDecisionTOS_MDL/TOS_20201112/TOS_2012080320/TOS/AEB/TOS_AEBJunct_20201208/AEBJunc_Object_Condition/AEBJA_TargetCondition/TOS_AEBJunc_TargetsCondition/AEBJunc_VehTargetCondition/Subsystem ==
  Object_MovingState : Inport
  Compare To Constant1 : simulink/Logic and Bit Operations/Compare To Constant  relop===  const=OFM_OBJ_MOVINGSTATE_E.MOVING  OutDataTypeStr=boolean
      settings: AttributesFormatString=%<const> = 2
  Compare To Constant2 : simulink/Logic and Bit Operations/Compare To Constant  relop===  const=OFM_OBJ_MOVINGSTATE_E.MOVING_SLOWLY  OutDataTypeStr=boolean
      settings: AttributesFormatString=%<const> = 5
  Data Type Conversion : DataTypeConversion  OutDataTypeStr=Enum: OFM_OBJ_MOVINGSTATE_E
  Logical Operator1 : Logic  Operator=OR  AllPortsSameDT=off  OutDataTypeStr=boolean
  TOS_AEBJuncVehTargetMovStateFlg : Outport
  wires:
  Compare To Constant1/1 -> Logical Operator1/1
  Logical Operator1/1 -> TOS_AEBJuncVehTargetMovStateFlg/1
  Compare To Constant2/1 -> Logical Operator1/2
  Object_MovingState/1 -> Data Type Conversion/1
  Data Type Conversion/1 -> Compare To Constant2/1, Compare To Constant1/1

== system PubIfDecisionTOS_MDL/TOS_20201112/TOS_2012080320/TOS/AEB/TOS_AEBJunct_20201208/AEBJunc_Object_Condition/AEBJA_TargetCondition/TOS_AEBJunc_TargetsCondition/AEBJunc_VehTargetCondition/TOS_AEBJunc_VehTargetMoveDir ==
  Object_Dx : Inport
  PP_ObjMovingDirSignalProcessing : Inport  Port=2
  Object_HeadingAngle : Inport  Port=3
  Object_VX : Inport  Port=4
  Object_VY : Inport  Port=5
  VIE_EgoVelocity : Inport  Port=6
  axvRefMs2 : Inport  Port=7
  AEBJunc_Target_ID_K1 : Inport  Port=8
  ObjectID : Inport  Port=9
  AEBJunc_TargetMovDirAborDly : Subsystem
  Abs : Abs
  Abs3 : Abs
  Add{,2..4} (4 alike) : Sum
  Add1 : Sum  Inputs=+-
  Compare To Constant : simulink/Logic and Bit Operations/Compare To Constant  relop=<  const=P_TOS_OncomingTarget_VxabsOffset_val  OutDataTypeStr=boolean
      settings: AttributesFormatString=%<const> = -0.7m/s
  Compare To Constant16 : simulink/Logic and Bit Operations/Compare To Constant  relop=>  const=P_TOS_ObjLatCroYawAngMaxThre_Val  OutDataTypeStr=boolean
      settings: AttributesFormatString=P_TOS_ObjLatCroYawAngMaxThre_Val = 135
  Compare To Constant2 : simulink/Logic and Bit Operations/Compare To Constant  relop===  const=ObjectMovingOrientation_E.OnComingDir  OutDataTypeStr=boolean
      settings: AttributesFormatString=%<const>
  Compare To Constant3 : simulink/Logic and Bit Operations/Compare To Constant  relop=>  const=P_TOS_ObjOncomingYawAngMaxThre_Val  OutDataTypeStr=boolean
      settings: AttributesFormatString=P_TOS_ObjOncomingYawAngMaxThre_Val = 180
  Compare To Constant4 : simulink/Logic and Bit Operations/Compare To Constant  relop=<  const=0  OutDataTypeStr=boolean
  Constant : Constant  Value=C_TOS_StepTime_Val
  Constant1 : Constant  Value=C_TOS_StepTime_Val
  Constant2 : Constant  Value=P_TOS_OncomingVehDxChangeOffset_Val
  Data Type Conversion2 : DataTypeConversion  OutDataTypeStr=Enum: ObjectMovingOrientation_E
  Gain : Gain  Gain=1/2
  Gain1 : Gain  Gain=1/2
  Logical Operator : Logic  Operator=OR  Inputs=4  AllPortsSameDT=off  OutDataTypeStr=boolean
  Logical Operator10 : Logic  AllPortsSameDT=off  OutDataTypeStr=boolean
  Logical Operator2 : Logic  AllPortsSameDT=off  OutDataTypeStr=boolean
  Logical Operator3 : Logic  AllPortsSameDT=off  OutDataTypeStr=boolean
  Math Function : Math  Operator=square  SaturateOnIntegerOverflow=on
  Product : Product
  Product1 : Product
  Relational Operator : RelationalOperator  Operator=>  OutDataTypeStr=boolean  RndMeth=Simplest
  Terminator : Terminator
  Unit Delay{,1..3} (4 alike) : UnitDelay  InitialCondition=255  SampleTime=-1  HasFrameUpgradeWarning=on
  TOS_AEBJuncVehTargetMovDirFlg : Outport
  wires:
  Logical Operator/1 -> AEBJunc_TargetMovDirAborDly/3(TOS_AEBJunc_MovDir_Flag)
  VIE_EgoVelocity/1 -> [VIE_EgoVelocity], Add/2
  Compare To Constant/1 -> Logical Operator/3
  PP_ObjMovingDirSignalProcessing/1 -> Data Type Conversion2/1
  Add/1 -> Compare To Constant/1
  Data Type Conversion2/1 -> Compare To Constant2/1
  Abs/1 -> Compare To Constant16/1, Compare To Constant3/1
  Logical Operator10/1 -> Logical Operator/2
  Compare To Constant16/1 -> Logical Operator10/1
  Object_VX/1 -> Add/1
  Compare To Constant2/1 -> Logical Operator/1
  Object_HeadingAngle/1 -> Abs/1
  Compare To Constant3/1 -> Logical Operator10/2
  Object_Dx/1 -> Add1/1, Unit Delay/1
  Unit Delay/1 -> Add1/2
  Add1/1 -> Compare To Constant4/1, Abs3/1
  Compare To Constant4/1 -> Logical Operator2/1
  Abs3/1 -> Relational Operator/1
  [VIE_EgoVelocity] -> Unit Delay2/1
  Constant/1 -> Product/2
  Constant1/1 -> Math Function/1
  Math Function/1 -> Product1/2
  Product1/1 -> Gain/1
  Gain/1 -> Add2/2
  Product/1 -> Add2/1
  axvRefMs2/1 -> Add3/1, Unit Delay1/1
  Add2/1 -> Add4/1
  Relational Operator/1 -> Unit Delay3/1, Logical Operator3/1
  Logical Operator2/1 -> Logical Operator/4
  Unit Delay1/1 -> Add3/2
  Add3/1 -> Gain1/1
  Gain1/1 -> Product1/1
  Unit Delay2/1 -> Product/1
  Constant2/1 -> Add4/2
  Add4/1 -> Relational Operator/2
  Unit Delay3/1 -> Logical Operator3/2
  Logical Operator3/1 -> Logical Operator2/2
  AEBJunc_TargetMovDirAborDly/1(TOS_AEBJunc_MovDirFlag_Delay) -> TOS_AEBJuncVehTargetMovDirFlg/1
  ObjectID/1 -> AEBJunc_TargetMovDirAborDly/2(ObjectID)
  AEBJunc_Target_ID_K1/1 -> AEBJunc_TargetMovDirAborDly/1(AEBJunc_Target_ID_K1)
  Object_VY/1 -> Terminator/1

== system PubIfDecisionTOS_MDL/TOS_20201112/TOS_2012080320/TOS/AEB/TOS_AEBJunct_20201208/AEBJunc_Object_Condition1/AEBJA_TargetCondition/TOS_AEBJunc_TargetsCondition/AEBJunc_PedTargetCondition/AEBJunc_PedTargetADxDyArea ==
  Object_Dx : Inport
  Object_Dy : Inport  Port=2
  Abs : Abs
  Compare To Constant1 : simulink/Logic and Bit Operations/Compare To Constant  relop=<=  const=C_TOS_AEBJAPedObjDxThre_Val  OutDataTypeStr=boolean
      settings: AttributesFormatString=C_TOS_AEBJAObjDxThre_Val = 25
  Compare To Constant2 : simulink/Logic and Bit Operations/Compare To Constant  relop=>  const=C_TOS_EgoDxRefPoint_m  OutDataTypeStr=boolean
      settings: AttributesFormatString=C_TOS_EgoDxRefPoint_m = 0
  Compare To Constant6 : simulink/Logic and Bit Operations/Compare To Constant  relop=<=  const=C_TOS_AEBJAPedObjDyThre_Val  OutDataTypeStr=boolean
      settings: AttributesFormatString=C_TOS_AEBJAObjDyThre_Val = 10 m
  Logical Operator : Logic  AllPortsSameDT=off  OutDataTypeStr=boolean
  Logical Operator1 : Logic  AllPortsSameDT=off  OutDataTypeStr=boolean
  TOS_AEBJunc_DxDyAreaFlag : Outport
  wires:
  Object_Dx/1 -> Compare To Constant2/1, Compare To Constant1/1
  Compare To Constant6/1 -> Logical Operator1/2
  Logical Operator1/1 -> TOS_AEBJunc_DxDyAreaFlag/1
  Compare To Constant2/1 -> Logical Operator/2
  Compare To Constant1/1 -> Logical Operator/1
  Abs/1 -> Compare To Constant6/1
  Object_Dy/1 -> Abs/1
  Logical Operator/1 -> Logical Operator1/1

== system PubIfDecisionTOS_MDL/TOS_20201112/TOS_2012080320/TOS/AEB/TOS_AEBJunct_20201208/AEBJunc_Object_Condition1/AEBJA_TargetCondition/TOS_AEBJunc_TargetsCondition/AEBJunc_PedTargetCondition/AEBJunc_PedTargetFusionTypeJudge ==
  PP_ObjFusType_FC_FR_Confirm : Inport
  PP_ObjFusType_FR_Confirm : Inport  Port=2
  Compare To Constant5 : simulink/Logic and Bit Operations/Compare To Constant  relop===  const=C_TOS_PP_ObjFusType_FC_FR_Confirm_b  OutDataTypeStr=boolean
      settings: AttributesFormatString=C_TOS_PP_ObjFusType_FC_FR_Confirm_b = 1
  Compare To Constant6 : simulink/Logic and Bit Operations/Compare To Constant  relop===  const=C_TOS_PP_ObjFusType_FR_Confirm_b  OutDataTypeStr=boolean
      settings: AttributesFormatString=C_TOS_PP_ObjFusType_FR_Confirm_b = 1
  Logical Operator : Logic  Operator=OR  AllPortsSameDT=off  OutDataTypeStr=boolean
  AEBJunc_TargetFusionTypeFlag : Outport
  wires:
  Logical Operator/1 -> AEBJunc_TargetFusionTypeFlag/1
  Compare To Constant5/1 -> Logical Operator/1
  Compare To Constant6/1 -> Logical Operator/2
  PP_ObjFusType_FC_FR_Confirm/1 -> Compare To Constant5/1
  PP_ObjFusType_FR_Confirm/1 -> Compare To Constant6/1

== system PubIfDecisionTOS_MDL/TOS_20201112/TOS_2012080320/TOS/AEB/TOS_AEBJunct_20201208/AEBJunc_Object_Condition1/AEBJA_TargetCondition/TOS_AEBJunc_TargetsCondition/AEBJunc_PedTargetCondition/AEBJunc_PedTargetMoveDir ==
  Object_Dy : Inport
  Object_Dx : Inport  Port=2
  PP_ObjMovingDirSignalProcessing : Inport  Port=3
  Object_HeadingAngle : Inport  Port=4
  Object_VX : Inport  Port=5
  Object_VY : Inport  Port=6
  VIE_EgoVelocity : Inport  Port=7
  axvRefMs2 : Inport  Port=8
  Bus Creator : BusCreator  Inputs=8
  Logical Operator : Logic  Operator=OR  AllPortsSameDT=off  OutDataTypeStr=boolean
  TOS_AEBJuncTargetCrossing : Subsystem
  TOS_AEBJuncTargetOncoming : Subsystem
  TOS_AEBJuncTargetMovDirFlg : Outport
  wires:
  Logical Operator/1 -> TOS_AEBJuncTargetMovDirFlg/1
  axvRefMs2/1 -> Bus Creator/8  "axvRefMs2"
  Object_Dx/1 -> Bus Creator/2  "Object_Dx"
  TOS_AEBJuncTargetOncoming/1(TOS_AEBJuncTargetOncomingFlg) -> Logical Operator/2
  TOS_AEBJuncTargetCrossing/1(TOS_AEBJuncTargetCrossingFlg) -> Logical Operator/1
  Bus Creator/1 -> TOS_AEBJuncTargetCrossing/1(Object_Infor), TOS_AEBJuncTargetOncoming/1(Object_Infor)
  Object_Dy/1 -> Bus Creator/1  "Object_Dy"
  Object_VY/1 -> Bus Creator/6  "Object_VY"
  VIE_EgoVelocity/1 -> Bus Creator/7  "VIE_EgoVelocity"
  Object_VX/1 -> Bus Creator/5  "Object_VX"
  Object_HeadingAngle/1 -> Bus Creator/4  "Object_HeadingAngle"
  PP_ObjMovingDirSignalProcessing/1 -> Bus Creator/3  "PP_ObjMovingDirSignalProcessing"

== system PubIfDecisionTOS_MDL/TOS_20201112/TOS_2012080320/TOS/AEB/TOS_AEBJunct_20201208/AEBJunc_Object_Condition1/AEBJA_TargetCondition/TOS_AEBJunc_TargetsCondition/AEBJunc_PedTargetCondition/AEBJunc_PedTargetObjectTypeFlag ==
  ObjectType : Inport
  AEBLat_Target_ID_K1 : Inport  Port=2
  ObjectID : Inport  Port=3
  AEBJunc_PedTargetObjectTypeAborDly : Subsystem
  Compare To Constant3 : simulink/Logic and Bit Operations/Compare To Constant  relop===  const=OFM_OBJ_TYPE_E.PEDESTRIAN  OutDataTypeStr=boolean
      settings: AttributesFormatString=%<const>
  Compare To Constant4 : simulink/Logic and Bit Operations/Compare To Constant  relop===  const=OFM_OBJ_TYPE_E.MOTORBIKE  OutDataTypeStr=boolean
      settings: AttributesFormatString=%<const>
  Compare To Constant5 : simulink/Logic and Bit Operations/Compare To Constant  relop===  const=OFM_OBJ_TYPE_E.BICYCLE  OutDataTypeStr=boolean
      settings: AttributesFormatString=%<const>
  Data Type Conversion : DataTypeConversion  OutDataTypeStr=Enum: OFM_OBJ_TYPE_E
  Logical Operator3 : Logic  Operator=OR  Inputs=3  AllPortsSameDT=off  OutDataTypeStr=boolean
  AEBJunc_PedTargetObjectTypeFlag : Outport
  wires:
  AEBJunc_PedTargetObjectTypeAborDly/1(TOS_AEBJunc_PedObjectTypeFilt) -> AEBJunc_PedTargetObjectTypeFlag/1
  AEBLat_Target_ID_K1/1 -> AEBJunc_PedTargetObjectTypeAborDly/1(AEBJunc_PedTarget_ID_K1)
  ObjectID/1 -> AEBJunc_PedTargetObjectTypeAborDly/2(ObjectID)
  Compare To Constant3/1 -> Logical Operator3/1
  Compare To Constant5/1 -> Logical Operator3/3
  Compare To Constant4/1 -> Logical Operator3/2
  Logical Operator3/1 -> AEBJunc_PedTargetObjectTypeAborDly/3(TOS_AEBJunc_PedObjectType)
  ObjectType/1 -> Data Type Conversion/1
  Data Type Conversion/1 -> Compare To Constant4/1, Compare To Constant5/1, Compare To Constant3/1

== system PubIfDecisionTOS_MDL/TOS_20201112/TOS_2012080320/TOS/AEB/TOS_AEBJunct_20201208/AEBJunc_Object_Condition1/AEBJA_TargetCondition/TOS_AEBJunc_TargetsCondition/AEBJunc_VehTargetCondition/AEBJunc_VehTargetADxDyArea ==
  Object_Dx : Inport
  Object_Dy : Inport  Port=2
  Abs : Abs
  Compare To Constant1 : simulink/Logic and Bit Operations/Compare To Constant  relop=<=  const=C_TOS_AEBJAVehObjDxThre_Val  OutDataTypeStr=boolean
      settings: AttributesFormatString=%<const> = 50
  Compare To Constant2 : simulink/Logic and Bit Operations/Compare To Constant  relop=>  const=C_TOS_EgoDxRefPoint_m  OutDataTypeStr=boolean
      settings: AttributesFormatString=C_TOS_EgoDxRefPoint_m = 0
  Compare To Constant6 : simulink/Logic and Bit Operations/Compare To Constant  relop=<=  const=C_TOS_AEBJAVehObjDyThre_Val  OutDataTypeStr=boolean
      settings: AttributesFormatString=C_TOS_AEBJAVehObjDyThre_Val = 10 m
  Logical Operator : Logic  AllPortsSameDT=off  OutDataTypeStr=boolean
  Logical Operator1 : Logic  AllPortsSameDT=off  OutDataTypeStr=boolean
  TOS_AEBJunc_VehDxDyAreaFlag : Outport
  wires:
  Logical Operator/1 -> Logical Operator1/1
  Object_Dy/1 -> Abs/1
  Abs/1 -> Compare To Constant6/1
  Compare To Constant1/1 -> Logical Operator/1
  Compare To Constant2/1 -> Logical Operator/2
  Logical Operator1/1 -> TOS_AEBJunc_VehDxDyAreaFlag/1
  Compare To Constant6/1 -> Logical Operator1/2
  Object_Dx/1 -> Compare To Constant1/1, Compare To Constant2/1

== system PubIfDecisionTOS_MDL/TOS_20201112/TOS_2012080320/TOS/AEB/TOS_AEBJunct_20201208/AEBJunc_Object_Condition1/AEBJA_TargetCondition/TOS_AEBJunc_TargetsCondition/AEBJunc_VehTargetCondition/AEBJunc_VehTargetFusionTypeJudge ==
  PP_ObjFusType_FC_FR_Confirm : Inport
  PP_ObjFusType_FR_Confirm : Inport  Port=2
  Compare To Constant5 : simulink/Logic and Bit Operations/Compare To Constant  relop===  const=C_TOS_PP_ObjFusType_FC_FR_Confirm_b  OutDataTypeStr=boolean
      settings: AttributesFormatString=C_TOS_PP_ObjFusType_FC_FR_Confirm_b = 1
  Compare To Constant6 : simulink/Logic and Bit Operations/Compare To Constant  relop===  const=C_TOS_PP_ObjFusType_FR_Confirm_b  OutDataTypeStr=boolean
      settings: AttributesFormatString=C_TOS_PP_ObjFusType_FR_Confirm_b = 1
  Logical Operator : Logic  Operator=OR  AllPortsSameDT=off  OutDataTypeStr=boolean
  AEBJunc_VehTargetFusionTypeFlag : Outport
  wires:
  PP_ObjFusType_FR_Confirm/1 -> Compare To Constant6/1
  PP_ObjFusType_FC_FR_Confirm/1 -> Compare To Constant5/1
  Compare To Constant6/1 -> Logical Operator/2
  Compare To Constant5/1 -> Logical Operator/1
  Logical Operator/1 -> AEBJunc_VehTargetFusionTypeFlag/1
